simulink model "Model_2022b"  (R2022b)
settings: Solver=VariableStepAuto  StartTime=0.0  StopTime=400  RelTol=1e-3
values from neighbouring files (symbols this model uses):
  Af = 2.46    [MainFile.m]
  Cd = 0.29    [MainFile.m]
  g = 9.81    [MainFile.m]
  m = X(i,1)    [MainFile.m]
  max_ac = 2    [MainFile.m]
  min_ac = -3    [MainFile.m]
  rho_air = 1.2256    [MainFile.m]
  slope = 0    [MainFile.m]
  standstill_distance = X(i,3)    [MainFile.m]
  time_gap = X(i,2)    [MainFile.m]
  v_ego = 22.22    [MainFile.m]
  verr_gain = 0.5    [MainFile.m]
  vx_gain = 0.4    [MainFile.m]
  x_ego = 0    [MainFile.m]
  xerr_gain = 0.2    [MainFile.m]
undefined symbols (not defined in the file or in its folder): magnitude
settings Model: Creator=Angelo  LastModifiedBy=Angelo

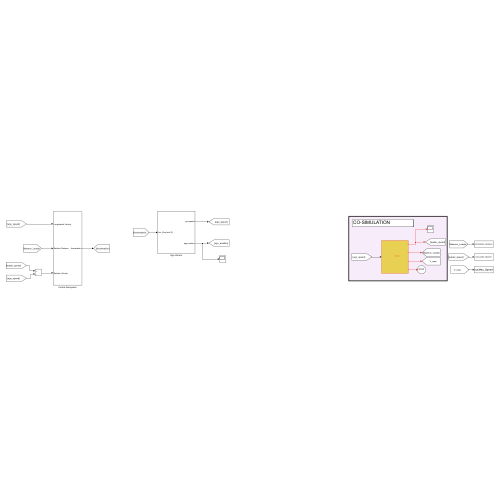
[thumbnail: Simulink's stored preview of the top-level diagram]
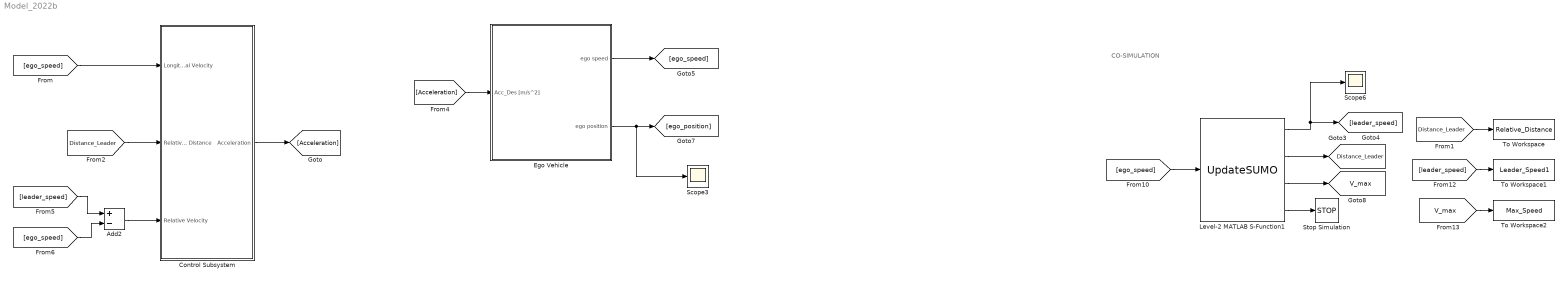
== system Model_2022b ==
  note: CO-SIMULATION
  Add2 : Sum  Inputs=+-
  Control Subsystem : Subsystem
  Ego Vehicle : Subsystem
  Level-2 MATLAB S-Function1 : M-S-Function  FunctionName=UpdateSUMO
      mask Display: image('C:\Users\Angelo\Desktop\UNIVERSITA\Progetti\2022_MEDIATOR\Test_CoSimulation\Examples\ACC\Images\SUMO.png'); % Use "Edit Image" on toolstrip to change.
  Scope3 : Scope
  Scope6 : Scope
  Stop Simulation : Stop
  To Workspace : ToWorkspace  VariableName=Relative_Distance  SampleTime=0.1
      settings: Save2DSignal=2-D array (concatenate along first dimension)
  To Workspace1 : ToWorkspace  VariableName=Leader_Speed1  SampleTime=0.1
      settings: Save2DSignal=2-D array (concatenate along first dimension)
  To Workspace2 : ToWorkspace  VariableName=Max_Speed  SampleTime=0.1
      settings: Save2DSignal=2-D array (concatenate along first dimension)
  tag scope: Distance_Leader=global, V_max=global
  wires:
  [Acceleration] -> Ego Vehicle/1(Acc_Des [m/s^2])
  Ego Vehicle/1(ego speed) -> [ego_speed]
  Ego Vehicle/2(ego position) -> [ego_position], Scope3/1
  Control Subsystem/1(Acceleration) -> [Acceleration]
  [ego_speed] -> Control Subsystem/1(Longitudinal Velocity)
  [Distance_Leader] -> Control Subsystem/2(Relative Distance)
  [ego_speed] -> Add2/2
  [leader_speed] -> Add2/1
  Add2/1 -> Control Subsystem/3(Relative Velocity)
  [leader_speed] -> To Workspace1/1
  Level-2 MATLAB S-Function1/3 -> [V_max]
  [V_max] -> To Workspace2/1
  Level-2 MATLAB S-Function1/2 -> [Distance_Leader]
  Level-2 MATLAB S-Function1/1 -> [leader_speed], Scope6/1
  Level-2 MATLAB S-Function1/4 -> Stop Simulation/1
  [Distance_Leader] -> To Workspace/1
  [ego_speed] -> Level-2 MATLAB S-Function1/1

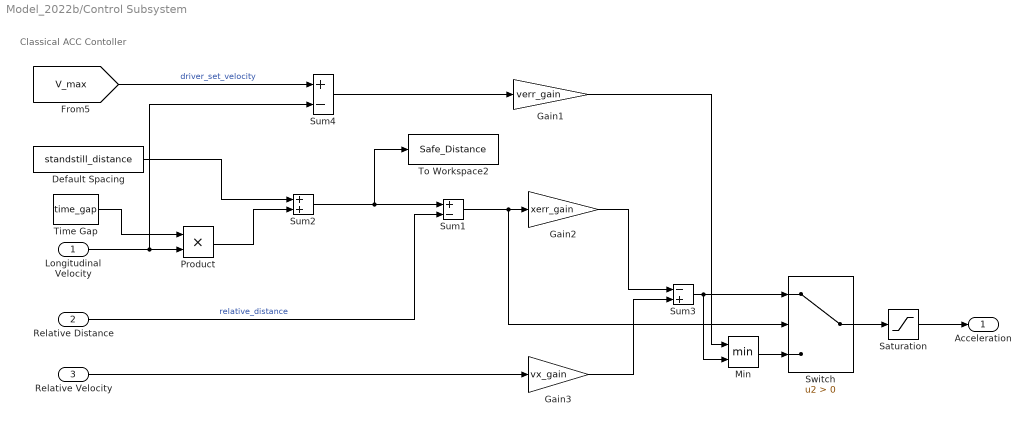
== system Model_2022b/Control Subsystem ==
  note: Classical ACC Contoller
  Longitudinal Velocity : Inport
  Relative Distance : Inport  Port=2
  Relative Velocity : Inport  Port=3
  Default Spacing : Constant  Value=standstill_distance  SampleTime=-1
  Gain1 : Gain  Gain=verr_gain
  Gain2 : Gain  Gain=xerr_gain
  Gain3 : Gain  Gain=vx_gain
  Min : MinMax  Inputs=2
  Product : Product
  Saturation : Saturate  UpperLimit=max_ac  LowerLimit=min_ac
  Sum1 : Sum  Inputs=+-
  Sum2 : Sum
  Sum3 : Sum  Inputs=-+
  Sum4 : Sum  Inputs=+-
  Switch : Switch  Criteria=u2 > Threshold  SaturateOnIntegerOverflow=off  InputSameDT=off
  Time Gap : Constant  Value=time_gap  SampleTime=-1
  To Workspace2 : ToWorkspace  VariableName=Safe_Distance  SampleTime=0.1
      settings: Save2DSignal=2-D array (concatenate along first dimension)
  Acceleration : Outport  VectorParamsAs1DForOutWhenUnconnected=off
  wires:
  Product/1 -> Sum2/2
  Switch/1 -> Saturation/1
  Sum1/1 -> Switch/2, Gain2/1
  Default Spacing/1 -> Sum2/1
  Min/1 -> Switch/3
  Gain3/1 -> Sum3/2
  [V_max] -> Sum4/1  "driver_set_velocity"
  Time Gap/1 -> Product/1
  Relative Velocity/1 -> Gain3/1
  Longitudinal Velocity/1 -> Product/2, Sum4/2
  Sum4/1 -> Gain1/1
  Saturation/1 -> Acceleration/1
  Relative Distance/1 -> Sum1/2  "relative_distance"
  Sum3/1 -> Min/2, Switch/1
  Gain1/1 -> Min/1
  Gain2/1 -> Sum3/1
  Sum2/1 -> To Workspace2/1, Sum1/1

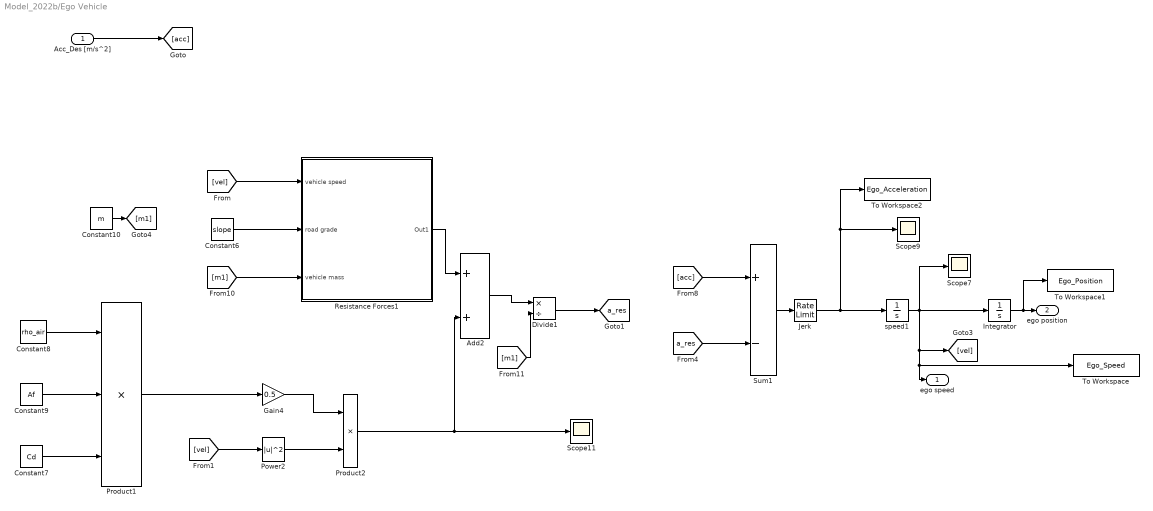
== system Model_2022b/Ego Vehicle ==
  Acc_Des [m/s^2] : Inport
  Add2 : Sum
  Constant10 : Constant  Value=m
  Constant6 : Constant  Value=slope
  Constant7 : Constant  Value=Cd
  Constant8 : Constant  Value=rho_air
  Constant9 : Constant  Value=Af
  Divide1 : Product  Inputs=*/
  Gain4 : Gain  Gain=0.5
  Integrator : Integrator  InitialCondition=x_ego
  Jerk : RateLimiter  RisingSlewLimit=15  FallingSlewLimit=-15
  Power2 : Math  Operator=magnitude^2  SignedPower=on
  Product1 : Product  Inputs=3
  Product2 : Product
  Resistance Forces1 : Subsystem
  Scope11 : Scope
  Scope7 : Scope
  Scope9 : Scope
  Sum1 : Sum  Inputs=+-
  To Workspace : ToWorkspace  VariableName=Ego_Speed  SampleTime=0.1
      settings: Save2DSignal=2-D array (concatenate along first dimension)
  To Workspace1 : ToWorkspace  VariableName=Ego_Position  SampleTime=0.1
      settings: Save2DSignal=2-D array (concatenate along first dimension)
  To Workspace2 : ToWorkspace  VariableName=Ego_Acceleration  SampleTime=0.1
      settings: Save2DSignal=2-D array (concatenate along first dimension)
  speed1 : Integrator  InitialCondition=v_ego  LimitOutput=on  UpperSaturationLimit=40  LowerSaturationLimit=0
  ego speed : Outport
  ego position : Outport  Port=2
  tag scope: a_res=global
  wires:
  Acc_Des [m/s^2]/1 -> [acc]
  Integrator/1 -> ego position/1, To Workspace1/1
  Resistance Forces1/1(Out1) -> Add2/1
  Product1/1 -> Gain4/1
  Constant8/1 -> Product1/1
  Jerk/1 -> To Workspace2/1, Scope9/1, speed1/1
  [m1] -> Resistance Forces1/3(vehicle mass)
  Constant9/1 -> Product1/2
  Constant10/1 -> [m1]
  [m1] -> Divide1/2
  Constant7/1 -> Product1/3
  Divide1/1 -> [a_res]
  Add2/1 -> Divide1/1
  Product2/1 -> Scope11/1, Add2/2
  speed1/1 -> Scope7/1, [vel], To Workspace/1, ego speed/1, Integrator/1
  [vel] -> Resistance Forces1/1(vehicle speed)
  Power2/1 -> Product2/2
  Sum1/1 -> Jerk/1
  [acc] -> Sum1/1
  [vel] -> Power2/1
  Gain4/1 -> Product2/1
  Constant6/1 -> Resistance Forces1/2(road grade)
  [a_res] -> Sum1/2

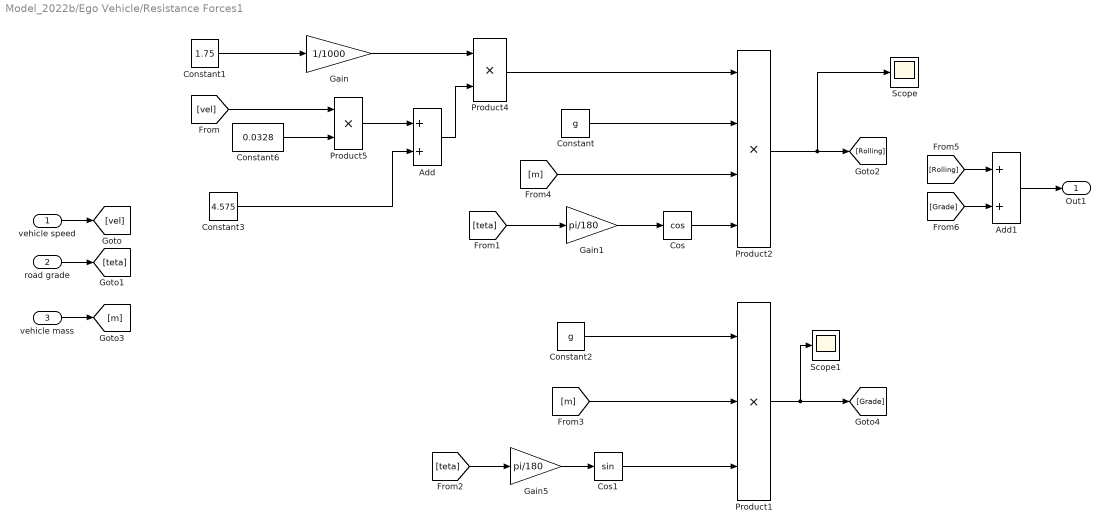
== system Model_2022b/Ego Vehicle/Resistance Forces1 ==
  vehicle speed : Inport
  road grade : Inport  Port=2
  vehicle mass : Inport  Port=3
  Add : Sum
  Add1 : Sum
  Constant : Constant  Value=g
  Constant1 : Constant  Value=1.75
  Constant2 : Constant  Value=g
  Constant3 : Constant  Value=4.575
  Constant6 : Constant  Value=0.0328
  Cos : Trigonometry  Operator=cos
  Cos1 : Trigonometry
  Gain : Gain  Gain=1/1000
  Gain1 : Gain  Gain=pi/180
  Gain5 : Gain  Gain=pi/180
  Product1 : Product  Inputs=3
  Product2 : Product  Inputs=4
  Product4 : Product
  Product5 : Product
  Scope : Scope
  Scope1 : Scope
  Out1 : Outport
  wires:
  Constant6/1 -> Product5/2
  Add/1 -> Product4/2
  Constant3/1 -> Add/2
  Gain/1 -> Product4/1
  Constant/1 -> Product2/2
  Product4/1 -> Product2/1
  Product5/1 -> Add/1
  [vel] -> Product5/1
  vehicle speed/1 -> [vel]
  Product2/1 -> Scope/1, [Rolling]
  [m] -> Product2/3
  Cos/1 -> Product2/4
  road grade/1 -> [teta]
  [teta] -> Gain1/1
  [teta] -> Gain5/1
  Cos1/1 -> Product1/3
  [m] -> Product1/2
  Product1/1 -> Scope1/1, [Grade]
  Constant2/1 -> Product1/1
  vehicle mass/1 -> [m]
  Add1/1 -> Out1/1
  [Rolling] -> Add1/1
  [Grade] -> Add1/2
  Gain5/1 -> Cos1/1
  Gain1/1 -> Cos/1
  Constant1/1 -> Gain/1
